simulink model "TrainSimulation"  (R2014a)
settings: Solver=ode45  StartTime=0.0  StopTime=100  RelTol=1e-3
values from neighbouring files (symbols this model uses):
  g = 9.8    [TrainSimulation_Run.m]
  k = 1    [TrainSimulation_Run.m]
  M1 = 1    [TrainSimulation_Run.m]
  M2 = 0.5    [TrainSimulation_Run.m]
  Mu = 0.02    [TrainSimulation_Run.m]
settings Model: Creator=DZR3QN  LastModifiedBy=DZR3QN

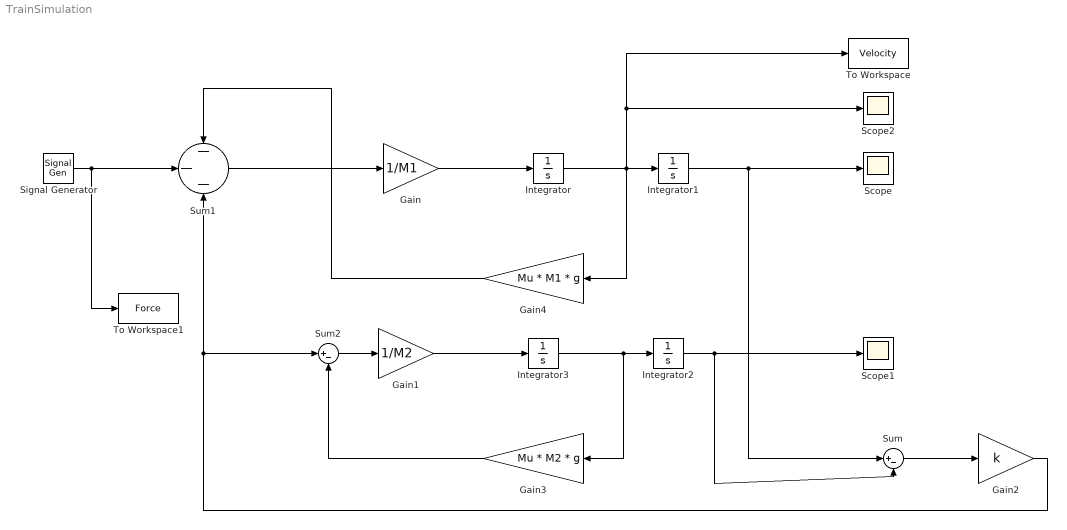
== system TrainSimulation ==
  Gain : Gain  Gain=1/M1
  Gain1 : Gain  Gain=1/M2
  Gain2 : Gain  Gain=k
  Gain3 : Gain  Gain=Mu * M2 * g
  Gain4 : Gain  Gain=Mu * M1 * g
  Integrator{,1..3} (4 alike) : Integrator
  Scope : Scope
  Scope1 : Scope
  Scope2 : Scope
      settings: SaveName=ScopeData2
  Signal Generator : SignalGenerator  WaveForm=square  Units=rad/sec
  Sum : Sum  Inputs=|+-
  Sum1 : Sum  Inputs=---
  Sum2 : Sum  Inputs=|+-
  To Workspace : ToWorkspace  VariableName=Velocity  SaveFormat=Timeseries  SampleTime=-1
  To Workspace1 : ToWorkspace  VariableName=Force  SaveFormat=Timeseries  SampleTime=-1
  wires:
  Gain/1 -> Integrator/1
  Gain1/1 -> Integrator3/1
  Integrator3/1 -> Gain3/1, Integrator2/1
  Integrator2/1 -> Sum/2, Scope1/1
  Integrator1/1 -> Sum/1, Scope/1
  Sum/1 -> Gain2/1
  Integrator/1 -> To Workspace/1, Scope2/1, Gain4/1, Integrator1/1
  Gain2/1 -> Sum2/1, Sum1/3
  Gain4/1 -> Sum1/1
  Sum1/1 -> Gain/1
  Sum2/1 -> Gain1/1
  Gain3/1 -> Sum2/2
  Signal Generator/1 -> Sum1/2, To Workspace1/1
